simulink model "scen3_PDproposed"  (R2022a)
settings: Solver=ode4  StartTime=0.0  StopTime=tsim*1.64  FixedStep=0.005  RelTol=1e-3
undefined symbols (not defined in the file): alpha, des_z, Kd, Kp, noise, peak_mp, Q, saturation_on, t_end_mp, trajectory
libraries: dspmtrx3 x2, dspindex x1
settings Model: Creator=PC  LastModifiedBy=PC
settings SolverCC: AlgebraicLoopSolver=TrustRegion
settings DataIOCC: ReturnWorkspaceOutputs=off
settings DebuggingCC: UnconnectedInputMsg=warning  UnconnectedOutputMsg=warning  UnconnectedLineMsg=warning  SFMachineParentedDataDiag=warning
settings RTWCC: DLArmComputeVersion=19.05

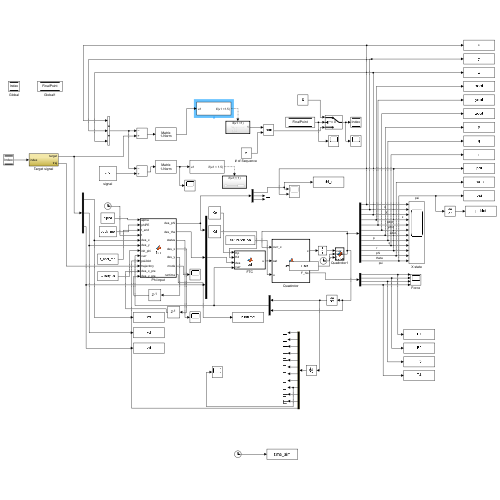
[thumbnail: Simulink's stored preview of the top-level diagram]
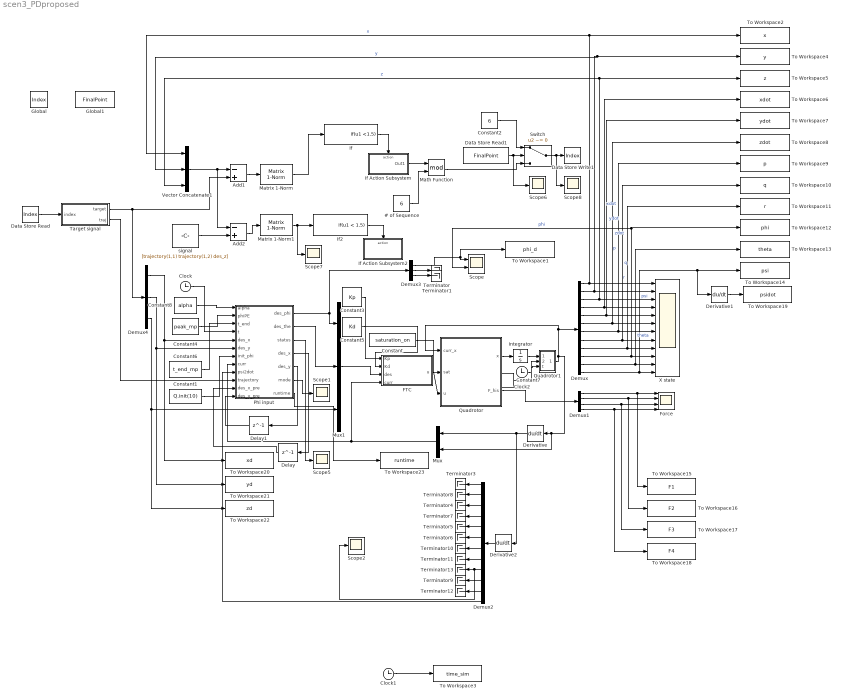
== system scen3_PDproposed ==
  "# of Sequence " : Constant  Value=6
  Add1 : Sum  Inputs=-+
  Add2 : Sum  Inputs=-+
  Clock : Clock
  Clock1 : Clock
  Clock2 : Clock
  Constant : Constant  Value=saturation_on
  Constant1 : Constant  Value=Q.init(10)
  Constant2 : Constant  Value=6
  Constant3 : Constant  Value=Kp
  Constant4 : Constant  Value=peak_mp
  Constant5 : Constant  Value=Kd
  Constant6 : Constant  Value=t_end_mp
  Constant7 : Constant  Value=noise
  Constant8 : Constant  Value=alpha
  Data Store Read : DataStoreRead  DataStoreName=Index  IndexOptions=Index vector (dialog)  Indices=1  OutputSizes=1
  Data Store Read1 : DataStoreRead  DataStoreName=FinalPoint  IndexOptions=Index vector (dialog)  Indices=1  OutputSizes=1
  Data Store Write1 : DataStoreWrite  DataStoreName=Index  IndexOptions=Index vector (dialog)  Indices=1  OutputSizes=1
  Delay : Delay  DelayLength=1
  Delay1 : Delay  DelayLength=1
  Demux : Demux  Outputs=12
  Demux1 : Demux
  Demux2 : Demux  Outputs=12
  Demux3 : Demux  Outputs=3
  Demux4 : Demux  Outputs=3
  Derivative : Derivative
  Derivative1 : Derivative
  Derivative2 : Derivative
  FTC : MATLAB Function  TreatAsAtomicUnit=on
  Force : Scope  NumInputPorts=4
  Global : DataStoreMemory  DataStoreName=Index  ReadBeforeWriteMsg=warning  WriteAfterWriteMsg=warning  WriteAfterReadMsg=warning  ShowAdditionalParam=off  OutDataTypeStr=double
  Global1 : DataStoreMemory  DataStoreName=FinalPoint  ReadBeforeWriteMsg=warning  WriteAfterWriteMsg=warning  WriteAfterReadMsg=warning  ShowAdditionalParam=off  OutDataTypeStr=double
  If : If  IfExpression=u1 <1.5  ShowElse=off
  If Action Subsystem : Subsystem  TreatAsAtomicUnit=on
  If Action Subsystem2 : Subsystem  TreatAsAtomicUnit=on
  If2 : If  IfExpression=u1 < 1.5  ShowElse=off
  Integrator : Integrator  InitialCondition=Q.init
  Math Function : Math  Operator=mod  SignedPower=on
  Matrix 1-Norm : dspmtrx3/Matrix  1-Norm  roundingMode=Floor  overflowMode=off  outputDataTypeStr=Inherit: Same as accumulator  outputMin=[]  outputMax=[]  outputLastDataTypeStr=Inherit: Same as accumulator
      settings: SourceProductBaseCode=DS
  Matrix 1-Norm1 : dspmtrx3/Matrix  1-Norm  roundingMode=Floor  overflowMode=off  outputDataTypeStr=Inherit: Same as accumulator  outputMin=[]  outputMax=[]  outputLastDataTypeStr=Inherit: Same as accumulator
      settings: SourceProductBaseCode=DS
  Mux : Mux  Inputs=2
  Mux1 : Mux  Inputs=3
  Phi input : MATLAB Function  TreatAsAtomicUnit=on
  Quadrotor : MATLAB Function  TreatAsAtomicUnit=on
  Quadrotor1 : MATLAB Function  TreatAsAtomicUnit=on
  Scope : Scope  NumInputPorts=2
  Scope{1..2,5..8} (6 alike) : Scope
  Switch : Switch  Criteria=u2 ~= 0  SaturateOnIntegerOverflow=off  InputSameDT=off
  Target signal : Subsystem
  Terminator{,1,3..13} (13 alike) : Terminator
  To Workspace1 : ToWorkspace  VariableName=phi_d  SampleTime=-1
      settings: Save2DSignal=2-D array (concatenate along first dimension)
  To Workspace10 : ToWorkspace  VariableName=q  SampleTime=-1
      settings: Save2DSignal=2-D array (concatenate along first dimension)
  To Workspace11 : ToWorkspace  VariableName=r  SampleTime=-1
      settings: Save2DSignal=2-D array (concatenate along first dimension)
  To Workspace12 : ToWorkspace  VariableName=phi  SampleTime=-1
      settings: Save2DSignal=2-D array (concatenate along first dimension)
  To Workspace13 : ToWorkspace  VariableName=theta  SampleTime=-1
      settings: Save2DSignal=2-D array (concatenate along first dimension)
  To Workspace14 : ToWorkspace  VariableName=psi  SampleTime=-1
      settings: Save2DSignal=2-D array (concatenate along first dimension)
  To Workspace15 : ToWorkspace  VariableName=F1  SampleTime=-1
      settings: Save2DSignal=2-D array (concatenate along first dimension)
  To Workspace16 : ToWorkspace  VariableName=F2  SampleTime=-1
      settings: Save2DSignal=2-D array (concatenate along first dimension)
  To Workspace17 : ToWorkspace  VariableName=F3  SampleTime=-1
      settings: Save2DSignal=2-D array (concatenate along first dimension)
  To Workspace18 : ToWorkspace  VariableName=F4  SampleTime=-1
      settings: Save2DSignal=2-D array (concatenate along first dimension)
  To Workspace19 : ToWorkspace  VariableName=psidot  SampleTime=-1
      settings: Save2DSignal=2-D array (concatenate along first dimension)
  To Workspace2 : ToWorkspace  VariableName=x  SampleTime=-1
      settings: Save2DSignal=2-D array (concatenate along first dimension)
  To Workspace20 : ToWorkspace  VariableName=xd  SampleTime=-1
      settings: Save2DSignal=2-D array (concatenate along first dimension)
  To Workspace21 : ToWorkspace  VariableName=yd  SampleTime=-1
      settings: Save2DSignal=2-D array (concatenate along first dimension)
  To Workspace22 : ToWorkspace  VariableName=zd  SampleTime=-1
      settings: Save2DSignal=2-D array (concatenate along first dimension)
  To Workspace23 : ToWorkspace  VariableName=runtime  SampleTime=-1
      settings: Save2DSignal=2-D array (concatenate along first dimension)
  To Workspace3 : ToWorkspace  VariableName=time_sim  SampleTime=-1
      settings: Save2DSignal=2-D array (concatenate along first dimension)
  To Workspace4 : ToWorkspace  VariableName=y  SampleTime=-1
      settings: Save2DSignal=2-D array (concatenate along first dimension)
  To Workspace5 : ToWorkspace  VariableName=z  SampleTime=-1
      settings: Save2DSignal=2-D array (concatenate along first dimension)
  To Workspace6 : ToWorkspace  VariableName=xdot  SampleTime=-1
      settings: Save2DSignal=2-D array (concatenate along first dimension)
  To Workspace7 : ToWorkspace  VariableName=ydot  SampleTime=-1
      settings: Save2DSignal=2-D array (concatenate along first dimension)
  To Workspace8 : ToWorkspace  VariableName=zdot  SampleTime=-1
      settings: Save2DSignal=2-D array (concatenate along first dimension)
  To Workspace9 : ToWorkspace  VariableName=p  SampleTime=-1
      settings: Save2DSignal=2-D array (concatenate along first dimension)
  Vector Concatenate1 : Concatenate  NumInputs=3
  X state : Scope  NumInputPorts=12
  signal : Constant  Value=[trajectory(1,1) trajectory(1,2) des_z]  VectorParams1D=off
  wires:
  Quadrotor/1(x) -> Integrator/1
  Mux1/1 -> FTC/3(des)
  Demux/3 -> To Workspace5/1, Vector Concatenate1/3, X state/3  "z"
  Demux/4 -> To Workspace6/1, X state/4  "xdot"
  Demux/5 -> To Workspace7/1, X state/5  "ydot"
  Demux/6 -> To Workspace8/1, X state/6  "zdot"
  Demux/7 -> To Workspace9/1, X state/7  "p"
  Demux/8 -> To Workspace10/1, X state/8  "q"
  Demux/9 -> To Workspace11/1, X state/9  "r"
  Demux/10 -> To Workspace12/1, Scope/2, X state/10  "phi"
  Demux/11 -> To Workspace13/1, X state/11  "theta"
  FTC/1(u) -> Quadrotor/3(u)
  Mux/1 -> FTC/4(curr), Phi input/8(curr)
  Derivative/1 -> Mux/1, Derivative2/1
  Clock/1 -> Phi input/4(t)
  Derivative2/1 -> Demux2/1
  Demux2/12 -> Phi input/9(psi2dot)
  Phi input/2(des_the) -> Mux1/2
  Demux2/1 -> Terminator3/1
  Demux2/2 -> Terminator8/1
  Demux2/3 -> Terminator4/1
  Demux2/4 -> Terminator7/1
  Demux2/5 -> Terminator5/1
  Demux2/6 -> Terminator6/1
  Demux2/10 -> Terminator9/1
  Demux2/7 -> Terminator10/1
  Demux2/8 -> Terminator11/1
  Demux2/11 -> Terminator12/1
  Demux2/9 -> Scope2/1, Terminator13/1
  Demux4/3 -> To Workspace22/1, Mux1/3
  Quadrotor/2(F_his) -> Demux1/1
  Demux1/1 -> To Workspace15/1, Force/1
  Demux1/3 -> To Workspace17/1, Force/3
  Demux1/4 -> To Workspace18/1, Force/4
  Demux1/2 -> Force/2, To Workspace16/1
  Clock1/1 -> To Workspace3/1
  Demux/12 -> Derivative1/1, To Workspace14/1, X state/12  "psi"
  Derivative1/1 -> To Workspace19/1
  Phi input/1(des_phi) -> Demux3/1, Mux1/1
  Demux3/1 -> To Workspace1/1, Scope/1
  Phi input/3(status) -> Scope5/1
  Constant/1 -> Quadrotor/2(sat)
  Data Store Read/1 -> Target signal/1(index)
  "# of Sequence "/1 -> Math Function/2
  Target signal/1(target) -> Demux4/1, Add1/2
  If Action Subsystem/1(Out1) -> Math Function/1
  Matrix 1-Norm/1 -> If/1
  Add1/1 -> Matrix 1-Norm/1
  Demux4/1 -> To Workspace20/1, Phi input/5("des_x ")
  Demux4/2 -> To Workspace21/1, Phi input/6("des_y ")
  Vector Concatenate1/1 -> Add2/1, Add1/1
  signal/1 -> Add2/2
  Matrix 1-Norm1/1 -> If2/1, Scope7/1
  Add2/1 -> Matrix 1-Norm1/1
  If2/1 -> If Action Subsystem2/Action
  Data Store Read1/1 -> Scope6/1, Switch/2
  Switch/1 -> Scope8/1, Data Store Write1/1
  Math Function/1 -> Switch/3
  Constant2/1 -> Switch/1
  Target signal/2(traj) -> Phi input/10(trajectory)
  Demux/2 -> Vector Concatenate1/2, To Workspace4/1, X state/2  "y"
  Demux/1 -> To Workspace2/1, Vector Concatenate1/1, X state/1  "x"
  Constant8/1 -> Phi input/1(alpha)
  Constant4/1 -> Phi input/2(phiPE)
  Constant6/1 -> Phi input/3(t_end)
  Constant1/1 -> Phi input/7(init_phi)
  Constant3/1 -> FTC/1(Kp)
  Constant5/1 -> FTC/2(Kd)
  Phi input/4(des_x) -> Delay/1
  Phi input/5(des_y) -> Delay1/1
  Delay/1 -> Phi input/11(des_x_pre)
  Delay1/1 -> Phi input/12(des_y_pre)
  Phi input/6(mode) -> Scope1/1
  If/1 -> If Action Subsystem/Action
  Demux3/2 -> Terminator/1
  Demux3/3 -> Terminator1/1
  Phi input/7(runtime) -> To Workspace23/1
  Quadrotor1/1(x) -> Mux/2, Derivative/1, Quadrotor/1(curr_x), Demux/1
  Integrator/1 -> Quadrotor1/1(curr_x)
  Constant7/1 -> Quadrotor1/2(noise)
  Clock2/1 -> Quadrotor1/3(t)

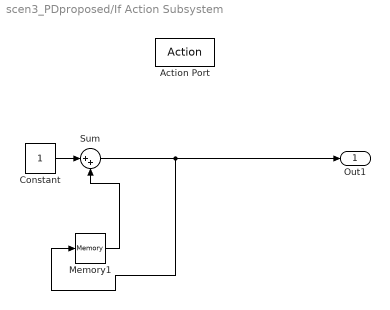
== system scen3_PDproposed/If Action Subsystem ==
  Action Port : ActionPort  ActionPortLabel=if(u1 <1)
  Constant : Constant
  Memory1 : Memory
  Sum : Sum  Inputs=|++
  Out1 : Outport  VectorParamsAs1DForOutWhenUnconnected=off
  wires:
  Memory1/1 -> Sum/2
  Constant/1 -> Sum/1
  Sum/1 -> Memory1/1, Out1/1

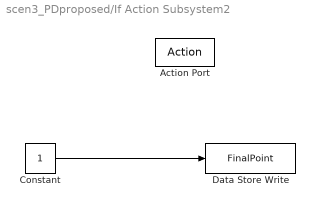
== system scen3_PDproposed/If Action Subsystem2 ==
  Action Port : ActionPort  ActionPortLabel=if(u1 < 1)
  Constant : Constant
  Data Store Write : DataStoreWrite  DataStoreName=FinalPoint  IndexOptions=Index vector (dialog)  Indices=1  OutputSizes=1
  wires:
  Constant/1 -> Data Store Write/1

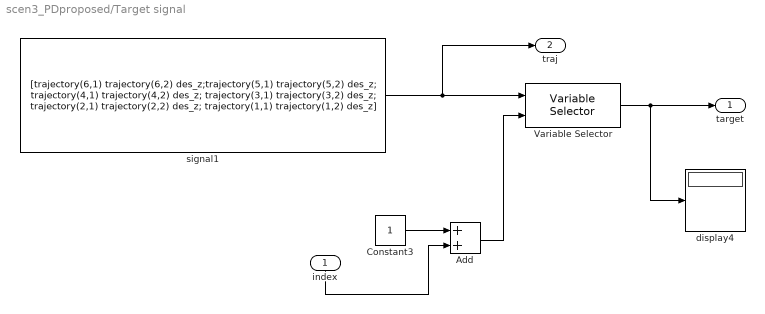
== system scen3_PDproposed/Target signal ==
  index : Inport
  Add : Sum
  Constant3 : Constant
  Variable Selector : dspindex/Variable Selector  NumInputs=1  rowsOrCols=Rows  IdxMode=Variable  Elements=[1 3]  ZerOneIdxMode=One-based  errmode=Clip Index  FillMode=on  FillValues=0
  display4 : Display
  signal1 : Constant  Value=[trajectory(6,1) trajectory(6,2) des_z;trajectory(5,1) trajectory(5,2) des_z; trajectory(4,1) trajectory(4,2) des_z; trajectory(3,1) trajectory(3,2) des_z; trajectory(2,1) trajectory(2,2) des_z; trajectory(1,1) trajectory(1,2) des_z]  VectorParams1D=off
  target : Outport  VectorParamsAs1DForOutWhenUnconnected=off
  traj : Outport  Port=2  VectorParamsAs1DForOutWhenUnconnected=off
  wires:
  Add/1 -> Variable Selector/2
  Variable Selector/1 -> target/1, display4/1
  index/1 -> Add/2
  signal1/1 -> traj/1, Variable Selector/1
  Constant3/1 -> Add/1

== matlab function scen3_PDproposed/Quadrotor1 ==
  settings: updateMethod=DISCRETE
  data: curr_x input; noise input; t input; x output
function x  = system(curr_x, noise, t)

ind = fix(t/0.01)+1;
mu = 0;
sigma = 0.01;


x = curr_x;
x(1) = curr_x(1)+noise(ind,1);
x(2) = curr_x(2)+noise(ind,2);
x(3) = curr_x(3)+noise(ind,3);

== matlab function scen3_PDproposed/Quadrotor ==
  settings: updateMethod=DISCRETE
  data: curr_x input; sat input; u input; x output; F_his output
function [x,F_his] = system(curr_x,sat,u)
% x = {xyz xyzvel pqr phi theta psi}
x = zeros(12,1);
% Properties
m = 1.282; g = 9.81;
Ix = 4.856*10^-3; Iy = Ix; Iz = 8.801*10^-3;
b = 0.0066;
kr = 0.02;
kt = 0.5;
l = 0.1;

u_temp = zeros(3,1);
u_temp = u;
u = u_temp;

T = u(1); tp = u(2); tq = u(3);% tr = u(4);
tr = b*(T-2*tp/l);
A = [1 1 1; 0 l 0;-l 0 l];

F=inv(A)*[T tp tq]';

f1 = F(1); f2 = F(2); f3 = F(3);
ub = m*g;
lb = 0;

saturation1_lb = 0;
saturation1_ub = 0;
saturation2_lb = 0;
saturation2_ub = 0;
saturation3_lb = 0;
saturation3_ub = 0;
saturation1_lb_margin = 0;
saturation1_ub_margin = 0;
saturation2_lb_margin = 0;
saturation2_ub_margin = 0;
saturation3_lb_margin = 0;
saturation3_ub_margin = 0;

if sat == 1
    if f1 < lb
        saturation1_lb = abs(lb - f1);
        saturation1_lb_margin = abs(lb - f1);
        f1 = lb;
    else
        saturation1_lb_margin = lb - f1;
    end
    
    if f1 > ub
        saturation1_ub = abs(ub - f1);
        saturation1_ub_margin = abs(ub - f1);
        f1 = ub;
    else
        saturation1_ub_margin = f1 - ub;
    end
    
    if f2 < lb
        saturation2_lb = abs(lb - f2);
        saturation2_lb_margin = abs(lb - f2);
        f2 = lb;
    else
        saturation2_lb_margin = lb - f2;
    end
    
    if f2 > ub
        saturation2_ub = abs(ub - f2);
        saturation2_ub_margin = abs(ub - f2);
        f2 = ub;
    else
        saturation2_ub_margin = f2 - ub;
    end
    
    if f3 < lb
        saturation3_lb = abs(lb - f3);
        saturation3_lb_margin = abs(lb - f3);
        f3 = lb;
    else
        saturation3_lb_margin = lb - f3;
    end
    
    if f3 > ub
        saturation3_ub = abs(ub - f3);
        saturation3_ub_margin = abs(ub - f3);
        f3 = ub;
    else
        saturation3_ub_margin = f3 - ub;
    end
end

saturation = max([saturation1_lb,saturation1_ub,saturation2_lb,saturation2_ub,saturation3_lb,saturation3_ub]);
saturation_margin = max([saturation1_lb_margin,saturation1_ub_margin,saturation2_lb_margin,saturation2_ub_margin,saturation3_lb_margin,saturation3_ub_margin]);

f4 = 0;
F_his = [f1 f2 f3 f4]';
T = f1+f2+f3;
tp = l*(f2);
tq = l*(f3-f1);
tr = b*(f1+f3-f2);

% Current state
x1  = curr_x(1);
x2  = curr_x(2);
x3  = curr_x(3);
x4  = curr_x(4);
x5  = curr_x(5);
x6  = curr_x(6);
x7  = curr_x(7);
x8  = curr_x(8);
x9  = curr_x(9);
x10 = curr_x(10);
x11 = curr_x(11);
x12 = curr_x(12);

% Position
x(1) = x4;
x(2) = x5;
x(3) = x6;
% Velocity
x(4) = T/m*(cos(x12)*sin(x11)*cos(x10) + sin(x12)*sin(x10)) - kt/m*x4;
x(5) = T/m*(sin(x12)*sin(x11)*cos(x10) - cos(x12)*sin(x10)) - kt/m*x5;
x(6) = -g + T*(1/m)*(cos(x10)*cos(x11)) - kt/m*x6;
% Body rate
x(7) = ((Ix-Iz)*x8*x9 + tp)/Ix;
x(8) = ((Iz-Ix)*x7*x9 + tq)/Ix;
x(9) = (-kr*x9 + tr)/Iz;
% Angle
x(10) = x7 + x8*sin(x10)*tan(x11) + x9*cos(x10)*tan(x11);
x(11) = x8*cos(x10) - x9*sin(x10);
x(12) = x8*sin(x10)/cos(x11) + x9*cos(x10)*cos(x11);

if x3<=0
    B=1;
else
    B=0;
end

== matlab function scen3_PDproposed/Phi input ==
  settings: updateMethod=DISCRETE
  data: alpha input; phiPE input; t_end input; des_phi output; des_the output; t input; des_x input; des_y input; init_phi input; curr input; psi2dot input; status output; trajectory input; des_x output; des_y output; des_x_pre input; des_y_pre input; mode output; runtime output
function [des_phi,des_the,status,des_x,des_y,mode,runtime]  = fcn(alpha,phiPE,t_end,t,des_x,des_y,init_phi,curr,psi2dot,trajectory,des_x_pre,des_y_pre)

tic;
m = 1.282; g = 9.81;
Ix = 4.856*10^-3; Iy = Ix; Iz = 8.801*10^-3;
b = 0.0066;
kr = 0.02; %drag coefficient
kt = 0.5;
l = 0.1;

phi0 = init_phi;
T = t_end;

rPE = (-kr/b+sqrt((kr/b)^2+8*m*g/(l*cos(phiPE))*(Iz-Iy)*tan(phiPE)))/(4*(Iz-Iy)*tan(phiPE)/l);
psidotPE = rPE*(tan(phiPE)*sin(phiPE)+cos(phiPE)); 
TPE = 2*pi/psidotPE;

phiPE2 = phiPE - alpha;
rPE2 = (-kr/b+sqrt((kr/b)^2+8*m*g/(l*cos(phiPE2))*(Iz-Iy)*tan(phiPE2)))/(4*(Iz-Iy)*tan(phiPE2)/l);
psidotPE2 = rPE2*(tan(phiPE2)*sin(phiPE2)+cos(phiPE2)); 
TPE2 = 2*pi/psidotPE2;

fPE2 = 1/TPE2;
fPE2 = fPE2*1.0004;
toff = 1/(4*fPE2);

a0 = phi0;
a1 = 0;
% a2 = 3*(b-init_phi)/t_end^2;
% a3 = -2*(b-init_phi)/t_end^3;
a2 = 0;
a3 = - (10*phi0 - 10*phiPE)/T^3;
a4 = (15*phi0 - 15*phiPE)/T^4;
a5 = -(6*phi0 - 6*phiPE)/T^5;

% current state
N = 0;
xdot   = curr(N+1); ydot   = curr(N+2); zdot   = curr(N+3);
x2dot  = curr(N+4); y2dot  = curr(N+5); z2dot  = curr(N+6);
pdot   = curr(N+7); qdot   = curr(N+8); rdot   = curr(N+9);
phidot = curr(N+10);thedot = curr(N+11);psidot = curr(N+12);

N = 12;
x    = curr(N+1); y    = curr(N+2); z    = curr(N+3);
xdot = curr(N+4); ydot = curr(N+5); zdot = curr(N+6);
p    = curr(N+7); q    = curr(N+8); r    = curr(N+9);
phi  = curr(N+10);the  = curr(N+11);psi  = curr(N+12);

while psi > pi
    psi = psi - 2*pi;
end

while psi < -pi
    psi = psi + 2*pi;
end

% corr_y = 0.73;
% corr_x = 0.54;

% for j = 1:7
%     tip_x = (trajectory(j,1)-trajectory(j-1,1));
%     tip_y = (trajectory(j,2)-trajectory(j-1,2));
%     
%     C_x = des_x + tip_x/100;
%     C_y = des_y + tip_y/100;
% end

R = 0.2016;
C_x = des_x;
C_y = des_y;
x_d = -R*sin(psi) + C_x; y_d = R*cos(psi) + C_y;
xdot_d = -R*cos(psi)*psidot; ydot_d = -R*sin(psi)*psidot;
x2dot_d = R*sin(psi)*psidot^2-R*cos(psi)*psi2dot; y2dot_d = R*cos(psi)*psidot^2-R*sin(psi)*psi2dot;

kpx = 10; kdx = 14;
kpx = 5; kdx = 25;
kpy = kpx; kdy = kdx;



persistent x0 y0 psi0 psi_LOS0 xPSMP yPSMP psiPSMP tPSMP tauPSMP t0
if isempty(x0)
    x0 = 0;
end
if isempty(y0)
    y0 = 0;
end
if isempty(psi0)
    psi0 = 0;
end
if isempty(psi_LOS0)
    psi_LOS0 = 0;
end
if isempty(xPSMP)
    xPSMP = 0;
end
if isempty(yPSMP)
    yPSMP = 0;
end
if isempty(psiPSMP)
    psiPSMP = 0;
end
if isempty(tPSMP)
    tPSMP = 0;
end
if isempty(tauPSMP)
    tauPSMP = 0;
end
if isempty(t0)
    t0 = 0;
end

data = [x0,y0,psi0,xPSMP,yPSMP,psiPSMP,psi_LOS0,tauPSMP,tPSMP];

delay_gain = 15;
    
% Obtained by ASMP,
% phi_hat = 0.6974;
% theta_hat = 0;
phi_d = 0;
phidot_d = 0;
phi2dot_d = 0;
phi_c = phi+phidot-(Iz-Ix)*r^2*tan(deg2rad(40))-2*(Iz-Ix)*r*tan(deg2rad(40))*rdot;
status = 1;

switch_psi = 0;
switch_pos = 0;



persistent switch_psi_occ
if isempty(switch_psi_occ)
    switch_psi_occ = 0;
end

persistent switch_pos_occ
if isempty(switch_pos_occ)
    switch_pos_occ = 0;
end

persistent mode_occ
if isempty(mode_occ)
    mode_occ = 0;
end

if des_x ~= des_x_pre || des_y ~= des_y_pre
    switch_pos_occ = 1;
end

mode = 0;

% Motion planner
if t <= t_end
    phi_d = a0 + a1*t + a2*t^2 + a3*t^3 + a4*t^4 + a5*t^5;
    phidot_d = a1 + 2*a2*t + 3*a3*t^2 + 4*a4*t^3 + 5*a5*t^4;
    phi2dot_d = 2*a2 + 6*a3*t + 12*a4*t^2 + 20*a5*t^3;
    mode = 1;
    mode_occ = 1;
elseif t <= t0+t_end*delay_gain
    phi_d = phiPE;
    phidot_d = 0;
    phi2dot_d = 0;
    x0 = x;
    y0 = y;
    psi0 = psi;
    psi_LOS0 = atan2(des_y-y0,des_x-x0);
    tauPSMP = (psi_LOS0-psi0-pi-psidotPE2*toff)/psidotPE + 0.03;
    while tauPSMP < 0
        tauPSMP = tauPSMP + TPE;
    end
    tPSMP = t0 + t_end*delay_gain + tauPSMP;
    mode = 2;
    mode_occ = 2;
elseif t <= t0+t_end*delay_gain + tauPSMP
    phi_d = phiPE;
    phidot_d = 0;
    phi2dot_d = 0;
    xPSMP = x;
    yPSMP = y;
    psiPSMP = psi;
    mode = 3;
    mode_occ = 3;
else % if switch_pos_occ == 1
    % PSMP
    phi_d = phiPE + alpha*(-sin(2*pi*fPE2*(t-1/(4*fPE2)-tPSMP)) - 1); % Down
    phidot_d = -2*alpha*pi*fPE2*cos(2*pi*fPE2*(t-1/(4*fPE2)-tPSMP));
    phi2dot_d = 4*alpha*(pi*fPE2)^2*sin(2*pi*fPE2*(t-1/(4*fPE2)-tPSMP));
    mode = 4;
    mode_occ = 4;
    if abs(phi_d - phiPE) < deg2rad(0.01) && switch_pos_occ == 1
        t0 = t;
        tauPSMP = 0;
        switch_pos_occ = 0;
        mode = 5;
        mode_occ = 5;
    end
% else
%     phi_d = phiPE + alpha*(-sin(2*pi*fPE2*(t-1/(4*fPE2)-tPSMP)) - 1); % Down
%     phidot_d = -2*alpha*pi*fPE2*cos(2*pi*fPE2*(t-1/(4*fPE2)-tPSMP));
%     phi2dot_d = 4*alpha*(pi*fPE2)^2*sin(2*pi*fPE2*(t-1/(4*fPE2)-tPSMP));
%     if abs(phi_d - phiPE) < deg2rad(1)
%         t0 = t;
%         tauPSMP = 0;
%         switch_pos_occ = 0;
%     end
%     mode = 5;
%     mode_occ = 5;
end




the_d = 0;    
thedot_d = 0;
the2dot_d = 0;
    

des_phi = [phi_d, phidot_d, phi2dot_d]';
des_the = [the_d, thedot_d, the2dot_d]';
runtime = toc;

== matlab function scen3_PDproposed/FTC ==
  data: Kp input; Kd input; des input; u output; curr input
function u = pd(Kp,Kd,des,curr)

m = 1.282; g = 9.81;
Ix = 4.856*10^-3; Iy = Ix; Iz = 8.801*10^-3;
b = 0.0066;
kr = 0.02;
kt = 0.5;
l = 0.1;

% current state
N = 0;
xdot   = curr(N+1); ydot   = curr(N+2); zdot   = curr(N+3);
x2dot  = curr(N+4); y2dot  = curr(N+5); z2dot  = curr(N+6);
pdot   = curr(N+7); qdot   = curr(N+8); rdot   = curr(N+9);
phidot = curr(N+10);thedot = curr(N+11);psidot = curr(N+12);

N = 12;
x    = curr(N+1); y    = curr(N+2); z    = curr(N+3);
xdot = curr(N+4); ydot = curr(N+5); zdot = curr(N+6);
p    = curr(N+7); q    = curr(N+8); r    = curr(N+9);
phi  = curr(N+10);the  = curr(N+11);psi  = curr(N+12);
des_temp = zeros(7,1);
des_temp = des;
des = des_temp;
% desired state
phi_d = des(1);
phidot_d = des(2);
phi2dot_d = des(3);
the_d = des(4);
thedot_d = des(5);
the2dot_d = des(6);
z_d   = des(7);

F = [p + q*sin(phi)*tan(the) + r*cos(phi)*tan(the)
     q*cos(phi) - r*sin(phi)
     -(Iz - Iy)*q*r/Ix
     -(Ix - Iz)*p*r/Iy
     -kr*r/Iz
     zdot
     -kt*zdot/m - g];
 
G = [0 0 0
     0 0 0
     0 1/Ix 0
     0 0 1/Iy
     b/Iz -2*b/(l*Iz) 0
     0 0 0
     cos(phi)*cos(the)/m 0 0];
 
J = [q*cos(phi)*tan(the)-r*sin(phi)*tan(the) q*sin(phi)*sec(the)^2+r*cos(phi)*sec(the)^2 1 sin(phi)*tan(the) cos(phi)*tan(the) 0 0
     -q*sin(phi)-r*cos(phi) 0 0 cos(phi) -sin(phi) 0 0
     0 0 0 0 0 0 1];

ubar = [phi2dot_d + Kp*(phi_d-phi) + Kd*(phidot_d-phidot)
        the2dot_d + Kp*(the_d-the) + Kd*(thedot_d-thedot)
        10*(z_d-z) + (0-zdot)];
    
u = inv(J*G)*(-J*F + ubar);
